simulink model "SpeedGoatSimulinkModel"  (R2019a)
settings: Solver=FixedStepDiscrete  StartTime=0.0  StopTime=21  RelTol=1e-3  EnableMultiTasking=on
values from neighbouring files (symbols this model uses):
  sF = 500    [createSineWaves.m]    (also in createSineWavesStim.m)
undefined symbols (not defined in the file or in its folder): IO397
libraries: speedgoatlib_fpga_analog_io x2, slrtlib x2, speedgoatlib_fpga x1
settings Model: ExtModeArchiveMode=auto  ExtModeArchiveFileName=SGOut  ExtModeArchiveDirName=D:\Simulink RT\SignalOutTest  Creator=BNL User  LastModifiedBy=BNL User
settings SolverCC: ConcurrentTasks=on  AutoInsertRateTranBlk=on
settings DataIOCC: SaveFormat=StructureWithTime  SignalLogging=off  DSMLogging=off
settings OptimizationCC: BlockReduction=off  OptimizeBlockIOStorage=off  BufferReuse=off  GlobalBufferReuse=off  ExpressionFolding=off  LocalBlockOutputs=off  OptimizeDataStoreBuffers=off  BusAssignmentInplaceUpdate=off
settings HardwareCC: ProdBitPerPointer=32  ProdBitPerSizeT=32  ProdBitPerPtrDiffT=32  ProdLargestAtomicFloat=None  ProdWordSize=32  ProdLongLongMode=on  ProdHWDeviceType=Generic->32-bit x86 compatible
settings RTWCC: SystemTargetFile=slrt.tlc  TemplateMakefile=slrt_default_tmf  Description=Simulink Real-Time  CodeExecutionProfiling=on  RTWCompilerOptimization=on
settings SimulinkRealTimeCC: SupportVariableSizeSignals=on  PreserveStateflowLocalDataDimensions=off  RL32LogTETModifier=off

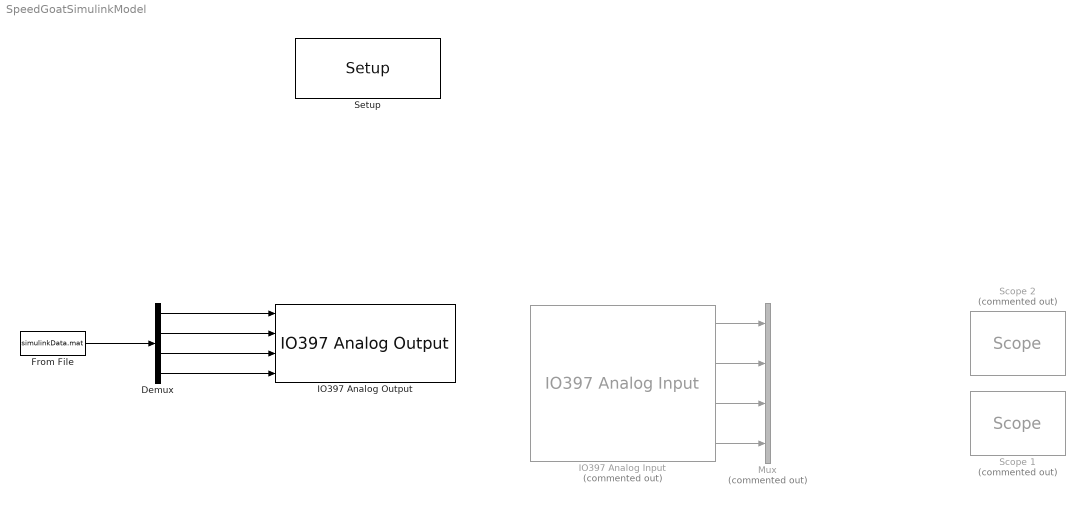
== system SpeedGoatSimulinkModel ==
  Demux : Demux
  From File : FromFile  FileName=simulinkData.mat  SampleTime=1/sF
  IO397 Analog Input : speedgoatlib_fpga_analog_io/IO397 Analog Input  Commented=on  id=1  chan=1:4  range=+5.12 V  trigger=Initiator  ts=1/500  pciSlot=-1  board=IO397-50k
      settings: SourceProductName=Simulink Real-Time: Speedgoat I/O Driver Library
  IO397 Analog Output : speedgoatlib_fpga_analog_io/IO397 Analog Output  id=1  chan=1:4  initVal=0  resetVal=0  ts=1/sF  pciSlot=-1  board=IO397-50k  span=+5
      settings: SourceProductName=Simulink Real-Time: Speedgoat Library
  Mux : Mux  Commented=on
  Scope 1 : slrtlib/Displays and Logging/Scope   Commented=on  scopeno=2  scopetype=Target  autostart=on  viewmode=Graphical sliding  formatstr='%15.6f'  grid=on  ylimits=[0,0]  nosamples=5000  noprepostsamples=0  interleave=1  triggermode=FreeRun  triggersignal=1  trigsignalfromport=off  triggerlevel=0.0  triggerslope=Either  triggerscope=1  triggersample=0  filename=data.dat  mode=Lazy  writesize=512  autorestart=off  dynamicfilemode=off  maxwritefilesize=512*1024^2
  Scope 2 : slrtlib/Displays and Logging/Scope   Commented=on  scopeno=1  scopetype=Target  autostart=on  viewmode=Graphical sliding  formatstr='%15.6f'  grid=on  ylimits=[0,0]  nosamples=5000  noprepostsamples=0  interleave=1  triggermode=FreeRun  triggersignal=1  trigsignalfromport=off  triggerlevel=0.0  triggerslope=Either  triggerscope=1  triggersample=0  filename=data.dat  mode=Lazy  writesize=512  autorestart=off  dynamicfilemode=off  maxwritefilesize=512*1024^2
  Setup : speedgoatlib_fpga/Setup/Setup  board=IO397-50k  id=1  frontIO=None  rearIO=None  bitstreamFile=speedgoat_IO397_50k_all_io  rev=1.0  timestamp_string=21/11/18 14:52:53  fpgaFreq=75 MHz  fpgaTick=13.3333 ns  ProgSpiFlash=off  ProgBPIFlash=off  pciSlot=-1  PullRPort0=pull-up 3.3V  VioPort0=3.3V  PullRPort1=pull-up 3.3V  VioPort1=3.3V  PullRPort2=pull-up 3.3V  VioPort2=3.3V  PullRPort3=pull-up 3.3V  VioPort3=3.3V  PullRPort4=pull-up 3.3V  VioPort4=3.3V  PullRPort5=pull-up 3.3V  VioPort5=3.3V  PullRPort6=pull-up 3.3V  VioPort6=3.3V  PullRPort15=pull-up 3.3V  PullRPort31=pull-up 3.3V  PullRPort47=pull-up 3.3V  PullRPort63=pull-up 3.3V
      settings: SourceProductName=Simulink Real-Time: Speedgoat Library
  wires:
  From File/1 -> Demux/1
  Demux/1 -> IO397 Analog Output/1
  Demux/2 -> IO397 Analog Output/2
  Demux/3 -> IO397 Analog Output/3
  Demux/4 -> IO397 Analog Output/4
  IO397 Analog Input/1 -> Mux/1
  IO397 Analog Input/2 -> Mux/2
  IO397 Analog Input/3 -> Mux/3
  IO397 Analog Input/4 -> Mux/4
